simulink model "room_model"  (R2017b)
settings: Solver=VariableStepAuto  StartTime=0.0  StopTime=23  RelTol=1e-3
settings Model: Creator=jim  LastModifiedBy=jim

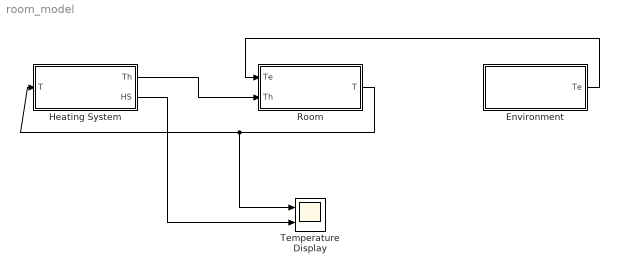
== system room_model ==
  Environment : Subsystem
  Heating System : Subsystem
  Room : Subsystem
  Temperature Display : Scope  NumInputPorts=2
  wires:
  Environment/1(Te) -> Room/1(Te)
  Room/1(T) -> Temperature Display/1, Heating System/1(T)
  Heating System/1(Th) -> Room/2(Th)
  Heating System/2(HS) -> Temperature Display/2

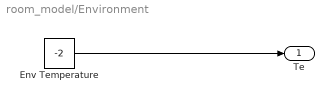
== system room_model/Environment ==
  Env Temperature : Constant  Value=-2
  Te : Outport
  wires:
  Env Temperature/1 -> Te/1

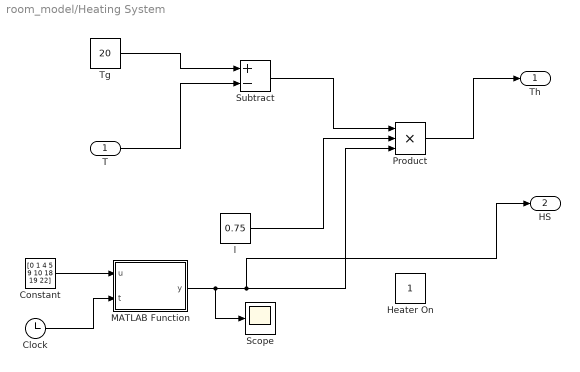
== system room_model/Heating System ==
  T : Inport
  Clock : Clock
  Constant : Constant  Value=[0 1 4 5 9 10 18 19 22]
  Heater On : Constant
  MATLAB Function : MATLAB Function  TreatAsAtomicUnit=on
  Product : Product  Inputs=3
  Scope : Scope
  Subtract : Sum  Inputs=+-
  Tg : Constant  Value=20
  l : Constant  Value=0.75
  Th : Outport
  HS : Outport  Port=2
  wires:
  Tg/1 -> Subtract/1
  T/1 -> Subtract/2
  Subtract/1 -> Product/1
  l/1 -> Product/2
  Product/1 -> Th/1
  Constant/1 -> MATLAB Function/1(u)
  Clock/1 -> MATLAB Function/2(t)
  MATLAB Function/1(y) -> Scope/1, HS/1, Product/3

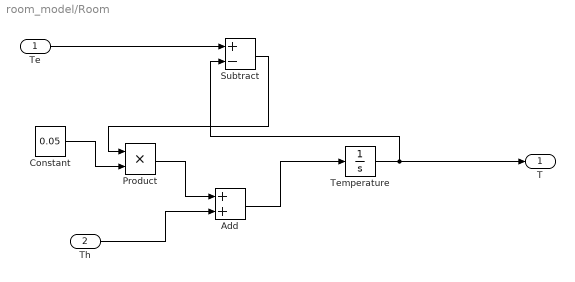
== system room_model/Room ==
  Te : Inport
  Th : Inport  Port=2
  Add : Sum
  Constant : Constant  Value=0.05
  Product : Product
  Subtract : Sum  Inputs=+-
  Temperature : Integrator  InitialCondition=10
  T : Outport
  wires:
  Th/1 -> Add/2
  Add/1 -> Temperature/1
  Temperature/1 -> Subtract/2, T/1
  Te/1 -> Subtract/1
  Constant/1 -> Product/2
  Subtract/1 -> Product/1
  Product/1 -> Add/1

== matlab function room_model/Heating System/MATLAB Function ==
  data: u input; y output; t input
function y = fcn(u, t)

time = int32(floor(t));
y = any(time==u);

end
